simulink model "kalman_filter_check"  (R2023a)
settings: Solver=FixedStepAuto  StartTime=0.0  StopTime=input_settings.flight_time  FixedStep=input_settings.dt  RelTol=1e-3
values from neighbouring files (symbols this model uses):
  reference_values_nonlinear = sensor_measurements(2,:)    [test_kalman_filter.m]
  Rn = eye(length(input_settings.sensors)) .* 1e-6    [evaluate_kf_design.m]
  sys_LQR = ss(sys_LQR.A, sys_LQR.B, sys_LQR.C(input_settings.sensors,:), sys_LQR.D(input_settings.sensors,:), input_settings.dt)    [test_kalman_filter.m]
undefined symbols (not defined in the file or in its folder): Discrete, sys_kf_new, Time
libraries: ctrlSharedLib x1
settings Model: Creator=sduess  LastModifiedBy=sduess

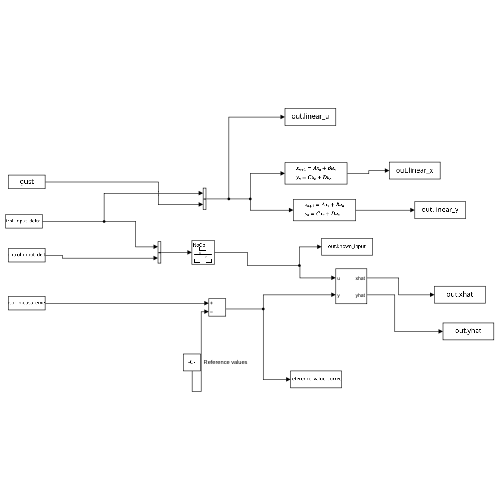
[thumbnail: Simulink's stored preview of the top-level diagram]
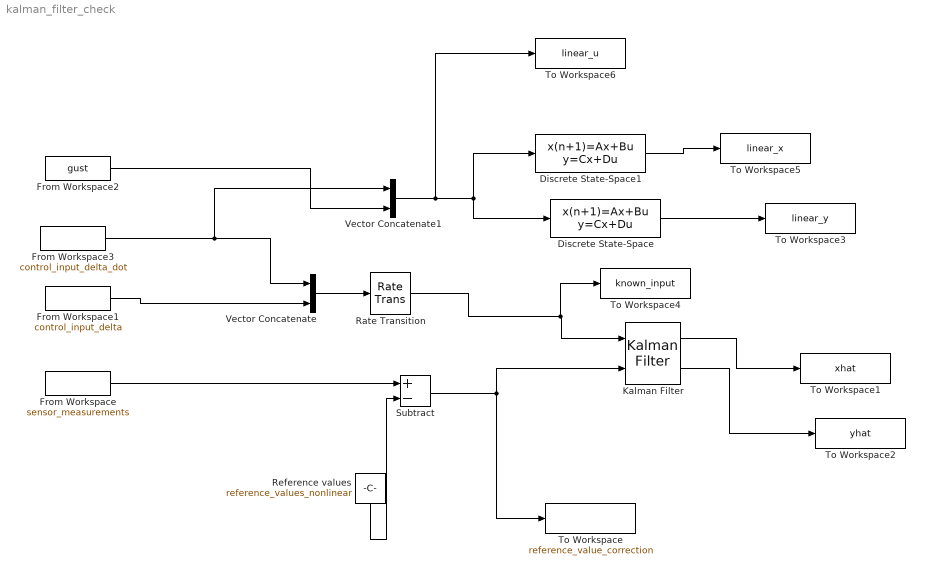
== system kalman_filter_check ==
  Discrete State-Space : DiscreteStateSpace  A=sys_LQR.A  B=sys_LQR.B  C=sys_LQR.C  D=sys_LQR.D  SampleTime=sys_LQR.Ts
  Discrete State-Space1 : DiscreteStateSpace  A=sys_LQR.A  B=sys_LQR.B  C=eye(size(sys_LQR.A))  D=sys_LQR.B.*0  SampleTime=sys_LQR.Ts
  From Workspace : FromWorkspace  VariableName=sensor_measurements  SampleTime=-1
  From Workspace1 : FromWorkspace  VariableName=control_input_delta  SampleTime=-1
  From Workspace2 : FromWorkspace  VariableName=gust
  From Workspace3 : FromWorkspace  VariableName=control_input_delta_dot  SampleTime=-1
  Kalman Filter : ctrlSharedLib/Kalman Filter  TimeDomain=Discrete-Time  UseCurrentEstimator=on  ModelSource=Individual A, B, C, D matrices  ModelSourceVariable=ss(0.95,1,1,0,1)  A=sys_kf_new.A  B=sys_kf_new.B(:,1:end-1)  C=sys_kf_new.C  D=sys_kf_new.D(:,1:end-1)  NumberOfStates=1  NumberOfInputs=1  NumberOfOutputs=1  InitialEstimateSource=Dialog  X0=0  P0=10  UseK=off  UseGH=on  NumberOfProcessNoiseInputs=1  G=[sys_kf_new.B(:,end) eye(size(sys_kf_new.B,1))]  TimeInvariantG=on  H="[sys_kf_new.D(:,end)  zeros(size(sys_kf_new.D(:,end),1), size(sys_kf_new.B,1))]"  TimeInvariantH=on  Q=Qn  TimeInvariantQ=on  R=Rn  TimeInvariantR=on  N=0  TimeInvariantN=on  AddInputPort=on  AddEnablePort=off  OutputEstimatedY=on  OutputP=off  Ts=-1
  Rate Transition : RateTransition  OutPortSampleTime=input_settings.dt
  Reference values : Constant  Value=reference_values_nonlinear
  Subtract : Sum  Inputs=+-
  To Workspace : ToWorkspace  VariableName=reference_value_correction  SaveFormat=Timeseries  SampleTime=-1
  To Workspace1 : ToWorkspace  VariableName=xhat  SaveFormat=Timeseries  SampleTime=-1
  To Workspace2 : ToWorkspace  VariableName=yhat  SaveFormat=Timeseries  SampleTime=-1
  To Workspace3 : ToWorkspace  VariableName=linear_y  SaveFormat=Timeseries  SampleTime=-1
  To Workspace4 : ToWorkspace  VariableName=known_input  SaveFormat=Timeseries  SampleTime=-1
  To Workspace5 : ToWorkspace  VariableName=linear_x  SaveFormat=Timeseries  SampleTime=-1
  To Workspace6 : ToWorkspace  VariableName=linear_u  SaveFormat=Timeseries  SampleTime=-1
  Vector Concatenate : Concatenate
  Vector Concatenate1 : Concatenate
  wires:
  Subtract/1 -> To Workspace/1, Kalman Filter/2
  Reference values/1 -> Subtract/2
  Kalman Filter/1 -> To Workspace1/1
  From Workspace1/1 -> Vector Concatenate/2
  From Workspace3/1 -> Vector Concatenate1/1, Vector Concatenate/1
  Vector Concatenate/1 -> Rate Transition/1
  Kalman Filter/2 -> To Workspace2/1
  From Workspace2/1 -> Vector Concatenate1/2
  Vector Concatenate1/1 -> To Workspace6/1, Discrete State-Space/1, Discrete State-Space1/1
  Discrete State-Space/1 -> To Workspace3/1
  Rate Transition/1 -> To Workspace4/1, Kalman Filter/1
  Discrete State-Space1/1 -> To Workspace5/1
  From Workspace/1 -> Subtract/1
